simulink library "cosineSquaredEnvironment_ul"  (R2018a)
settings: Solver=VariableStepAuto  StartTime=0.0  StopTime=10.0  RelTol=1e-3
values from neighbouring files (symbols this model uses):
  maxSteadySpeed_mPs = 1    [cosineSquaredEnvironment_init.m]
settings Model: Creator=mcobb  LastModifiedBy=mcobb

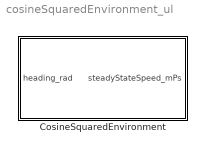
== system cosineSquaredEnvironment_ul ==
  CosineSquaredEnvironment : Subsystem

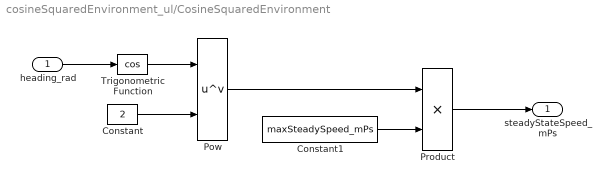
== system cosineSquaredEnvironment_ul/CosineSquaredEnvironment ==
  heading_rad : Inport
  Constant : Constant  Value=2
  Constant1 : Constant  Value=maxSteadySpeed_mPs
  Pow : Math  Operator=pow  RndMeth=Zero  SaturateOnIntegerOverflow=on
  Product : Product
  Trigonometric Function : Trigonometry  Operator=cos
  steadyStateSpeed_mPs : Outport
  wires:
  heading_rad/1 -> Trigonometric Function/1
  Trigonometric Function/1 -> Pow/1
  Constant/1 -> Pow/2
  Pow/1 -> Product/1
  Product/1 -> steadyStateSpeed_mPs/1
  Constant1/1 -> Product/2
